simulink model "NPV_Calculation"  (R2014a)
settings: Solver=ode45  StartTime=0.0  StopTime=1  RelTol=1e-3
libraries: simulink x1
settings Model: Creator=User  LastModifiedBy=User

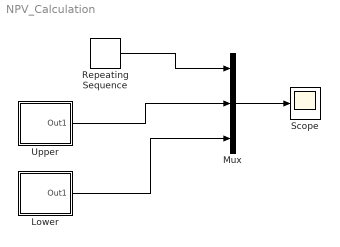
== system NPV_Calculation ==
  Lower : Subsystem
  Mux : Mux  Inputs=3
  Repeating Sequence : simulink/Sources/Repeating Sequence  rep_seq_t=[0 0.1 0.2]  rep_seq_y=[450 -450 450]
  Scope : Scope
  Upper : Subsystem
  wires:
  Mux/1 -> Scope/1
  Repeating Sequence/1 -> Mux/1
  Upper/1(Out1) -> Mux/2
  Lower/1(Out1) -> Mux/3

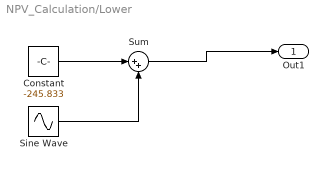
== system NPV_Calculation/Lower ==
  Constant : Constant  Value=-245.833
  Sine Wave : Sin  Amplitude=100  Frequency=2*pi*1  Phase=pi  SampleTime=0
  Sum : Sum  Inputs=|++
  Out1 : Outport
  wires:
  Sine Wave/1 -> Sum/2
  Sum/1 -> Out1/1
  Constant/1 -> Sum/1

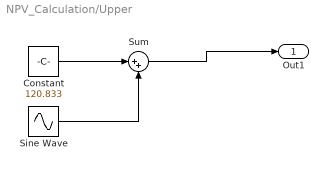
== system NPV_Calculation/Upper ==
  Constant : Constant  Value=120.833
  Sine Wave : Sin  Amplitude=225  Frequency=2*pi*1  SampleTime=0
  Sum : Sum  Inputs=|++
  Out1 : Outport
  wires:
  Constant/1 -> Sum/1
  Sum/1 -> Out1/1
  Sine Wave/1 -> Sum/2
